simulink model "BLDC_LADRC_Motor_Speed_Control"  (R2022b)
settings: Solver=ode4  StartTime=0.0  StopTime=2  FixedStep=1e-6  RelTol=1e-3
model workspace (MAT data in the model file):
  Ctrol_Mode = 1
  Current_Control_Mode = 2
  Current_PID_Upper_Limit = 1
  PWM_Period = 0.0001
  Speed_I = 10
  Speed_P = 10
  Speed_PID_Upper_Limit = 0.02
  Ts_time = 1e-06
  Wc = 1000
  Wo = 4000
  b0 = 300
  current_I = 1
  current_P = 100
  r = 80
undefined symbols (not defined in the file): sigbuilder_block
libraries: simulink x11, dsparch4 x6, spsSeriesRLCBranchLib x2, spsPermanentMagnetSynchronousMachineLib x1, spsCurrentMeasurementLib x1, spsDCVoltageSourceLib x1, slctrlblks x1, slpidlib x1, eePwmGenerator x1, spsTwoLevelConverterLib x1, spspowerguiLib x1
settings Model: Creator=31904  LastModifiedBy=31904

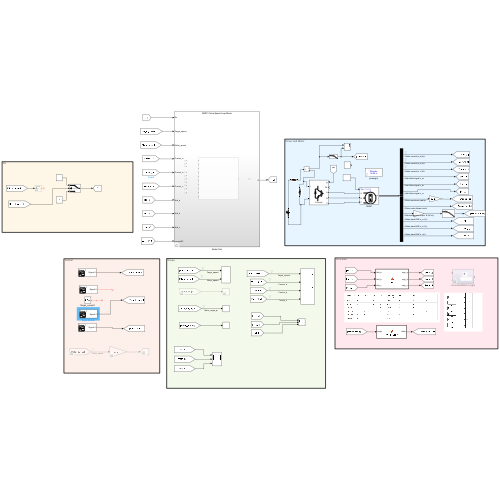
[thumbnail: Simulink's stored preview of the top-level diagram]
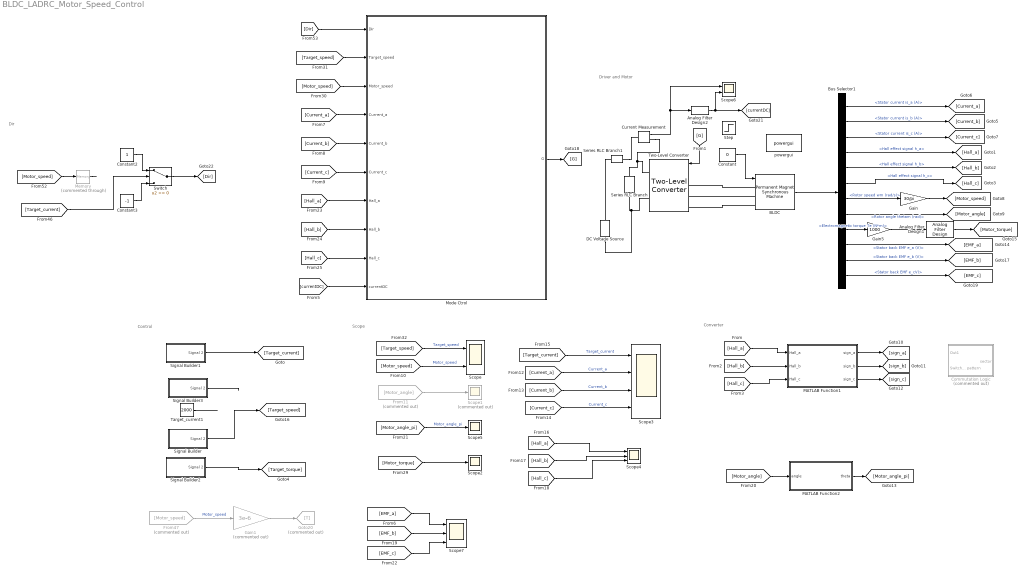
== system BLDC_LADRC_Motor_Speed_Control ==
  note: Dir
  note: Converter
  note: Control
  note: Scope
  note: Driver and Motor
  Analog Filter Design1 : dsparch4/Analog Filter Design  method=Butterworth  filttype=Lowpass  N=1  Wlo=1e2  Whi=80  Rp=2  Rs=40
  Analog Filter Design2 : dsparch4/Analog Filter Design  method=Butterworth  filttype=Lowpass  N=1  Wlo=100  Whi=80  Rp=2  Rs=40
  BLDC : spsPermanentMagnetSynchronousMachineLib/Permanent Magnet Synchronous Machine  NbPhases=3  FluxDistribution=Trapezoidal  RotorType=Round  MechanicalLoad=Torque Tm  PresetModel=No  ShowDetailedParameters=on  MeasurementBus=off  Resistance=1.005  Inductance=66e-6  dqInductances=[8.5e-3,8.5e-3]  La=0.0004  MachineConstant=Torque Constant (N.m / A_peak)  Flux=0.00785  VoltageCst=3.2882  TorqueCst=0.0314  Flat=120  Mechanical=[3e-05 0 2 0]  PolePairs=4  InitialConditions=[0,0, 0,0]  InitialConditions5ph=[0 0 0 0 0 0]  RefAngle=Aligned with phase A axis (original Park)  IterativeDiscreteModel=Trapezoidal non iterative  TsBlock=-1  TsPowergui=0
  Bus Selector1 : BusSelector  OutputSignals=Stator current is_a (A),Stator current is_b (A),Stator current is_c (A),Hall effect signal h_a,Hall effect signal h_b,Hall effect signal h_c,Rotor speed wm (rad/s),Rotor angle thetam (rad),Electromagnetic torque Te (N*m),Stator back EMF e_a (V),Stator back EMF e_b (V),Stator back EMF e_cV)
  Commutation Logic : Subsystem  Commented=on
  Constant : Constant  Value=0
  Constant2 : Constant
  Constant3 : Constant  Value=-1
  Current Measurement : spsCurrentMeasurementLib/Current Measurement  PhasorSimulation=off  OutputType=Complex  PSBequivalent=0
  DC Voltage Source : spsDCVoltageSourceLib/DC Voltage Source  Amplitude=28  Measurements=None
  From11 : From  Commented=on  GotoTag=Motor_angle
  From47 : From  Commented=on  GotoTag=Motor_speed
  Gain : Gain  Gain=30/pi
  Gain1 : Gain  Commented=on  Gain=3e-6
  Gain5 : Gain  Gain=1000
  Goto20 : Goto  Commented=on  GotoTag=T
  MATLAB Function1 : MATLAB Function  TreatAsAtomicUnit=on
  MATLAB Function2 : MATLAB Function  TreatAsAtomicUnit=on
  Memory : Memory  Commented=through
  Mode Ctrol : Subsystem  Variant=on
  Scope : Scope  NumInputPorts=2
  Scope1 : Scope  Commented=on
  Scope2 : Scope
  Scope3 : Scope  NumInputPorts=4
  Scope4 : Scope  NumInputPorts=3
  Scope5 : Scope
  Scope6 : Scope  NumInputPorts=2
  Scope7 : Scope  NumInputPorts=3
  Series RLC Branch : spsSeriesRLCBranchLib/Series RLC Branch  LConnTagsString=__new0  RConnTagsString=__new0  BranchType=C  Resistance=1  Inductance=1e-3  SetiL0=off  InitialCurrent=0  Capacitance=1e-6  Setx0=off  InitialVoltage=0  Measurements=None
  Series RLC Branch1 : spsSeriesRLCBranchLib/Series RLC Branch  LConnTagsString=__new0  RConnTagsString=__new0  BranchType=R  Resistance=1  Inductance=1e-3  SetiL0=off  InitialCurrent=0  Capacitance=1e-6  Setx0=off  InitialVoltage=0  Measurements=None
  Signal Builder : Subsystem  Tag=STV Subsys  LoadFcn=sigbuilder_block('load');  StartFcn=sigbuilder_block('start');  StopFcn=sigbuilder_block('stop');  ClipboardFcn=sigbuilder_block('clipboard');  mask(Sigbuilder block){tuvar=[0:10]}
      mask help: Simulink:masks:SigbuilderBlock_MD
      mask init:
      | if ~strcmp(get_param(bdroot(gcbh),'SimulationStatus'),'stopped') tuvar = sigbuilder_block('maskInit'); end
      settings: CopyFcn=sigbuilder_block('copy');  DeleteFcn=sigbuilder_block('delete');  ModelCloseFcn=sigbuilder_block('modelClose');  PreSaveFcn=sigbuilder_block('preSave');  PauseFcn=sigbuilder_block('pause');  ContinueFcn=sigbuilder_block('continue');  NameChangeFcn=sigbuilder_block('namechange');  OpenFcn=sigbuilder_block('open',[3234.3 -525.9 550.8 400.2 ]);  CloseFcn=sigbuilder_block('close');
      mask Display: plot(0, 0, 100, 100,[2, 2, 32, 32, 2], [68, 8, 8, 68, 68],[32, 2], [38, 38], [32, 19, 2],[53, 60, 44], [32, 17, 17, 2],[16, 16, 31, 31]);txt = getActiveGroup(gcbh);text(2, 100, txt,'verticalAlignment', 'top');
  Signal Builder1 : Subsystem  Tag=STV Subsys  LoadFcn=sigbuilder_block('load');  StartFcn=sigbuilder_block('start');  StopFcn=sigbuilder_block('stop');  ClipboardFcn=sigbuilder_block('clipboard');  mask(Sigbuilder block){tuvar=[0:10]}
      mask help: Simulink:masks:SigbuilderBlock_MD
      mask init:
      | if ~strcmp(get_param(bdroot(gcbh),'SimulationStatus'),'stopped') tuvar = sigbuilder_block('maskInit'); end
      settings: CopyFcn=sigbuilder_block('copy');  DeleteFcn=sigbuilder_block('delete');  ModelCloseFcn=sigbuilder_block('modelClose');  PreSaveFcn=sigbuilder_block('preSave');  PauseFcn=sigbuilder_block('pause');  ContinueFcn=sigbuilder_block('continue');  NameChangeFcn=sigbuilder_block('namechange');  OpenFcn=sigbuilder_block('open',[281.4 79.2 550.8 400.2 ]);  CloseFcn=sigbuilder_block('close');
      mask Display: plot(0, 0, 100, 100,[2, 2, 32, 32, 2], [68, 8, 8, 68, 68],[32, 2], [38, 38], [32, 19, 2],[53, 60, 44], [32, 17, 17, 2],[16, 16, 31, 31]);txt = getActiveGroup(gcbh);text(2, 100, txt,'verticalAlignment', 'top');
  Signal Builder2 : Subsystem  Tag=STV Subsys  LoadFcn=sigbuilder_block('load');  StartFcn=sigbuilder_block('start');  StopFcn=sigbuilder_block('stop');  ClipboardFcn=sigbuilder_block('clipboard');  mask(Sigbuilder block){tuvar=[0:10]}
      mask help: Simulink:masks:SigbuilderBlock_MD
      mask init:
      | if ~strcmp(get_param(bdroot(gcbh),'SimulationStatus'),'stopped') tuvar = sigbuilder_block('maskInit'); end
      settings: CopyFcn=sigbuilder_block('copy');  DeleteFcn=sigbuilder_block('delete');  ModelCloseFcn=sigbuilder_block('modelClose');  PreSaveFcn=sigbuilder_block('preSave');  PauseFcn=sigbuilder_block('pause');  ContinueFcn=sigbuilder_block('continue');  NameChangeFcn=sigbuilder_block('namechange');  OpenFcn=sigbuilder_block('open',[281.4 79.2 550.8 400.2 ]);  CloseFcn=sigbuilder_block('close');
      mask Display: plot(0, 0, 100, 100,[2, 2, 32, 32, 2], [68, 8, 8, 68, 68],[32, 2], [38, 38], [32, 19, 2],[53, 60, 44], [32, 17, 17, 2],[16, 16, 31, 31]);txt = getActiveGroup(gcbh);text(2, 100, txt,'verticalAlignment', 'top');
  Signal Builder3 : Subsystem  Tag=STV Subsys  LoadFcn=sigbuilder_block('load');  StartFcn=sigbuilder_block('start');  StopFcn=sigbuilder_block('stop');  ClipboardFcn=sigbuilder_block('clipboard');  mask(Sigbuilder block){tuvar=[0:10]}
      mask help: Simulink:masks:SigbuilderBlock_MD
      mask init:
      | if ~strcmp(get_param(bdroot(gcbh),'SimulationStatus'),'stopped') tuvar = sigbuilder_block('maskInit'); end
      settings: CopyFcn=sigbuilder_block('copy');  DeleteFcn=sigbuilder_block('delete');  ModelCloseFcn=sigbuilder_block('modelClose');  PreSaveFcn=sigbuilder_block('preSave');  PauseFcn=sigbuilder_block('pause');  ContinueFcn=sigbuilder_block('continue');  NameChangeFcn=sigbuilder_block('namechange');  OpenFcn=sigbuilder_block('open',[281.4 79.2 550.8 400.2 ]);  CloseFcn=sigbuilder_block('close');
      mask Display: plot(0, 0, 100, 100,[2, 2, 32, 32, 2], [68, 8, 8, 68, 68],[32, 2], [38, 38], [32, 19, 2],[53, 60, 44], [32, 17, 17, 2],[16, 16, 31, 31]);txt = getActiveGroup(gcbh);text(2, 100, txt,'verticalAlignment', 'top');
  Step : Step  Time=0  After=0.0005  SampleTime=0
  Switch : Switch  SaturateOnIntegerOverflow=off  InputSameDT=off
  Target_current1 : Constant  Value=2000
  Two-Level Converter : spsTwoLevelConverterLib/Two-Level Converter  ModelType=Switching devices  Ron=0.0001  Rs=1e6  Cs=inf  Vforward=[0,0]  Ron_Diode=1e-3  Rs_Diode=1e6  Cs_Diode=inf  Vf_Diode=1e-3  Rs_CurrentSource=inf  Ron_ACsource=1e-3
  powergui : spspowerguiLib/powergui  Priority=1  SimulationMode=Discrete  SampleTime=0.000001  frequency=60  Iterations=50  frequencyindice=0  Pbase=100e6  ErrMax=1e-4  UnitsV=kV  UnitsW=MW  buscounter=0  FunctionMessages=off  echomessages=off  EnableUseOfTLC=off  CurrentSourceSwitches=off  DisableSnubberDevices=off  DisableRonSwitches=off  DisableVfSwitches=off  DisplayEquations=off  AutomaticDiscreteSolvers=off  SolverType=Tustin/Backward Euler (TBE)  Interpol=off  ExternalGateDelay=off  methode=off  Ts=100  x0status=blocks  SPID=on  SwTol=0  HookPort=off  NonlinearTolerance=1e-4  nMaxIteration=100  ContinueOnMaxIteration=off  RestoreLinks=warning  ResistiveCurrentMeasurement=off  Frange=[0:2:500]  Ylog=off  Xlog=on  ShowGrid=off  save=off  variable=ZData  structure=0  ZoomFFT=off  StartTime=0.0  cycles=1  DisplayStyle=1  fundamental=60  FreqAxis=off  MaxFrequency=1000  frequencyindicesteady=1  RmsSteady=1  display=off
  wires:
  [G] -> Two-Level Converter/1
  Bus Selector1/3 -> [Current_c]  "<Stator current is_c (A)>"
  Bus Selector1/8 -> [Motor_angle]  "<Rotor angle thetam (rad)>"
  Bus Selector1/1 -> [Current_a]  "<Stator current is_a (A)>"
  Bus Selector1/6 -> [Hall_c]  "<Hall effect signal h_c>"
  Bus Selector1/4 -> [Hall_a]  "<Hall effect signal h_a>"
  Bus Selector1/2 -> [Current_b]  "<Stator current is_b (A)>"
  Bus Selector1/7 -> Gain/1  "<Rotor speed wm (rad/s)>"
  Bus Selector1/5 -> [Hall_b]  "<Hall effect signal h_b>"
  [Hall_a] -> MATLAB Function1/1(Hall_a)
  [Hall_b] -> MATLAB Function1/2(Hall_b)
  [Hall_c] -> MATLAB Function1/3(Hall_c)
  MATLAB Function1/1(sign_a) -> [sign_a]
  MATLAB Function1/2(sign_b) -> [sign_b]
  MATLAB Function1/3(sign_c) -> [sign_c]
  [Motor_speed] -> Scope/2  "Motor_speed"
  [Current_a] -> Scope3/2  "Current_a"
  [Current_b] -> Scope3/3  "Current_b"
  [Current_c] -> Scope3/4  "Current_c"
  [Target_current] -> Scope3/1  "Target_current"
  [Hall_a] -> Scope4/1
  [Hall_b] -> Scope4/2
  [Hall_c] -> Scope4/3
  From11/1 -> Scope1/1
  [Motor_angle] -> MATLAB Function2/1(angle)
  [Motor_angle_pi] -> Scope5/1  "Motor_angle_pi"
  MATLAB Function2/1(theta) -> [Motor_angle_pi]
  Bus Selector1/9 -> Gain5/1  "<Electromagnetic torque Te (N*m)>"
  [Motor_torque] -> Scope2/1
  [Target_speed] -> Scope/1  "Target_speed"
  Mode Ctrol/1(G) -> [G]
  [Target_speed] -> Mode Ctrol/2(Target_speed)
  [Motor_speed] -> Mode Ctrol/3(Motor_speed)
  [Current_a] -> Mode Ctrol/4(Current_a)
  [Current_b] -> Mode Ctrol/5(Current_b)
  [Current_c] -> Mode Ctrol/6(Current_c)
  Gain/1 -> [Motor_speed]
  Bus Selector1/10 -> [EMF_a]  "<Stator back EMF e_a (V)>"
  Bus Selector1/11 -> [EMF_b]  "<Stator back EMF e_b (V)>"
  Bus Selector1/12 -> [EMF_c]  "<Stator back EMF e_cV)>"
  [EMF_a] -> Scope7/1
  [EMF_b] -> Scope7/2
  [EMF_c] -> Scope7/3
  [Hall_a] -> Mode Ctrol/7(Hall_a)
  [Hall_b] -> Mode Ctrol/8(Hall_b)
  [Hall_c] -> Mode Ctrol/9(Hall_c)
  From47/1 -> Gain1/1  "Motor_speed"
  Gain1/1 -> Goto20/1
  BLDC/1 -> Bus Selector1/1
  Constant2/1 -> Switch/1
  Constant3/1 -> Switch/3
  Switch/1 -> [Dir]
  [Dir] -> Mode Ctrol/1(Dir)
  Gain5/1 -> Analog Filter Design1/1
  Signal Builder/1(Signal 2) -> [Target_speed]
  Constant/1 -> BLDC/1
  Current Measurement/1 -> Scope6/1, Analog Filter Design2/1
  Analog Filter Design2/1 -> [currentDC], Scope6/2
  [currentDC] -> Mode Ctrol/10(currentDC)
  [Motor_speed] -> Memory/1
  Memory/1 -> ?
  [Target_current] -> Switch/2
  Signal Builder1/1(Signal 2) -> [Target_current]
  Analog Filter Design1/1 -> [Motor_torque]
  Signal Builder2/1(Signal 2) -> [Target_torque]
  Target_current1/1 -> ?
  Signal Builder3/1(Signal 2) -> ?
  connections:
  DC Voltage Source/LConn1 -- Series RLC Branch/RConn1 -- Two-Level Converter/RConn2
  BLDC/LConn1 -- Two-Level Converter/LConn1
  BLDC/LConn2 -- Two-Level Converter/LConn2
  BLDC/LConn3 -- Two-Level Converter/LConn3
  Current Measurement/RConn1 -- Series RLC Branch/LConn1 -- Two-Level Converter/RConn1
  Series RLC Branch1/LConn1 -- DC Voltage Source/RConn1
  Series RLC Branch1/RConn1 -- Current Measurement/LConn1

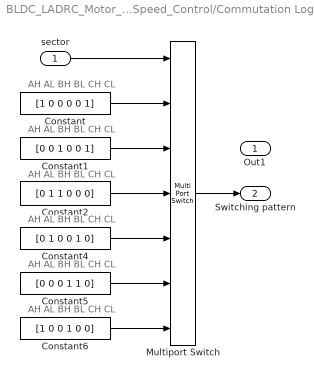
== system BLDC_LADRC_Motor_Speed_Control/Commutation Logic ==
  note: AH AL BH BL CH CL
  note: AH AL BH BL CH CL
  note: AH AL BH BL CH CL
  note: AH AL BH BL CH CL
  note: AH AL BH BL CH CL
  note: AH AL BH BL CH CL
  sector : Inport
  Constant : Constant  Value=[1 0 0 0 0 1]
  Constant1 : Constant  Value=[0 0 1 0 0 1]
  Constant2 : Constant  Value=[0 1 1 0 0 0]
  Constant4 : Constant  Value=[0 1 0 0 1 0]
  Constant5 : Constant  Value=[0 0 0 1 1 0]
  Constant6 : Constant  Value=[1 0 0 1 0 0]
  Multiport Switch : MultiPortSwitch  Inputs=6  SaturateOnIntegerOverflow=off  InputSameDT=off
  Out1 : Outport
  "  Switching pattern" : Outport  Port=2  VectorParamsAs1DForOutWhenUnconnected=off
  wires:
  Constant4/1 -> Multiport Switch/5
  Constant5/1 -> Multiport Switch/6
  Constant6/1 -> Multiport Switch/7
  sector/1 -> Multiport Switch/1
  Constant2/1 -> Multiport Switch/4
  Multiport Switch/1 -> "  Switching pattern"/1
  Constant1/1 -> Multiport Switch/3
  Constant/1 -> Multiport Switch/2

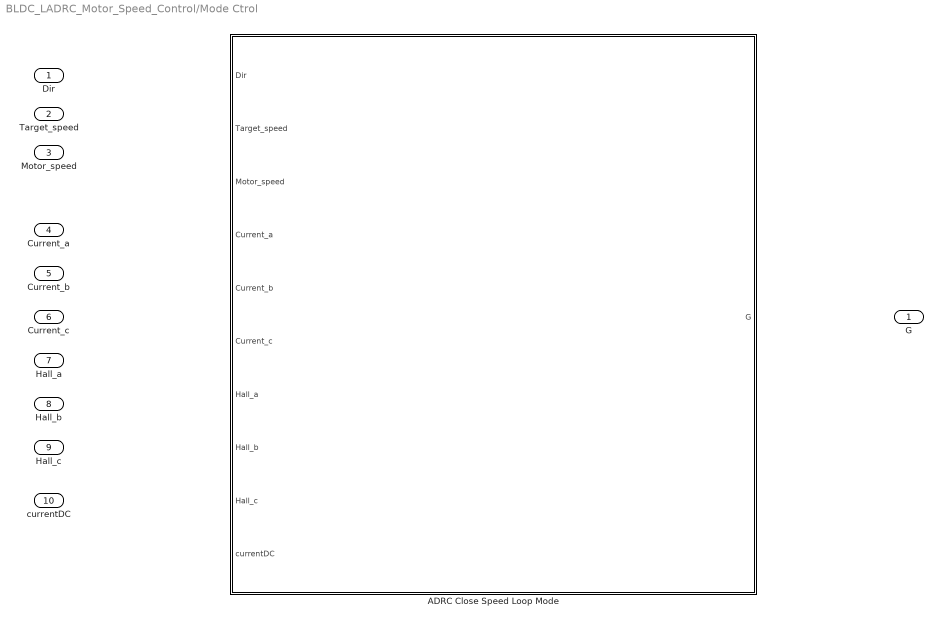
== system BLDC_LADRC_Motor_Speed_Control/Mode Ctrol ==
  Dir : Inport
  Target_speed : Inport  Port=2
  Motor_speed : Inport  Port=3
  Current_a : Inport  Port=4
  Current_b : Inport  Port=5
  Current_c : Inport  Port=6
  Hall_a : Inport  Port=7
  Hall_b : Inport  Port=8
  Hall_c : Inport  Port=9
  currentDC : Inport  Port=10
  ADRC Close Speed Loop Mode : Subsystem  TreatAsAtomicUnit=on  VariantControl=Ctrol_Mode==1
  G : Outport

== system BLDC_LADRC_Motor_Speed_Control/Signal Builder ==
  Demux : Demux  Tag=STV Demux  Outputs=1
      settings: DisplayOption=none
  FromWs : FromWorkspace  Tag=STV FromWs  VariableName=tuvar
      SigBuilderData=|
      | common.afterFinalStr = 'Extrapolate'
      | common.sampleTime = 0
      | dataSet.timeRange = [0 2]
      | dataSet.name = 'Group 1'
      | sbobj.Groups.Name = 'Group 1'
      | sbobj.Groups.Signals.Name = 'Signal 2'
      | sbobj.Groups.Signals.XData = [0 0.4 0.4 0.8 0.8 1.2 1.2 1.6 1.6 2]
      | sbobj.Groups.Signals.YData = [1000 1000 220 220 2000 2000 0 0 3000 3000]
      | sbobj.Groups.TimeRange = [0 2]
  Signal 2 : Outport  Tag=STV Outport
  wires:
  FromWs/1 -> Demux/1
  Demux/1 -> Signal 2/1

== system BLDC_LADRC_Motor_Speed_Control/Signal Builder1 ==
  Demux : Demux  Tag=STV Demux  Outputs=1
      settings: DisplayOption=none
  FromWs : FromWorkspace  Tag=STV FromWs  VariableName=tuvar
      SigBuilderData=|
      | common.afterFinalStr = 'Extrapolate'
      | common.sampleTime = 0
      | dataSet.timeRange = [0 10]
      | dataSet.name = 'Group 1'
      | sbobj.Groups.Name = 'Group 1'
      | sbobj.Groups.Signals.Name = 'Signal 2'
      | sbobj.Groups.Signals.XData = [0 0.2 0.2 0.4 0.4 10]
      | sbobj.Groups.Signals.YData = [1 1 -1 -1 0 0]
      | sbobj.Groups.TimeRange = [0 10]
  Signal 2 : Outport  Tag=STV Outport
  wires:
  Demux/1 -> Signal 2/1
  FromWs/1 -> Demux/1

== system BLDC_LADRC_Motor_Speed_Control/Signal Builder2 ==
  Demux : Demux  Tag=STV Demux  Outputs=1
      settings: DisplayOption=none
  FromWs : FromWorkspace  Tag=STV FromWs  VariableName=tuvar
      SigBuilderData=|
      | common.afterFinalStr = 'Extrapolate'
      | common.sampleTime = 0
      | dataSet.timeRange = [0 10]
      | dataSet.name = 'Group 1'
      | sbobj.Groups.Name = 'Group 1'
      | sbobj.Groups.Signals.Name = 'Signal 2'
      | sbobj.Groups.Signals.XData = [0 0.2 0.2 0.4 0.4 0.6 10]
      | sbobj.Groups.Signals.YData = [10 10 -10 -10 0 0 0]
      | sbobj.Groups.TimeRange = [0 10]
  Signal 2 : Outport  Tag=STV Outport
  wires:
  Demux/1 -> Signal 2/1
  FromWs/1 -> Demux/1

== system BLDC_LADRC_Motor_Speed_Control/Signal Builder3 ==
  Demux : Demux  Tag=STV Demux  Outputs=1
      settings: DisplayOption=none
  FromWs : FromWorkspace  Tag=STV FromWs  VariableName=tuvar
      SigBuilderData=|
      | common.afterFinalStr = 'Extrapolate'
      | common.sampleTime = 0
      | dataSet.timeRange = [0 0.5]
      | dataSet.name = 'Group 1'
      | sbobj.Groups.Name = 'Group 1'
      | sbobj.Groups.Signals.Name = 'Signal 2'
      | sbobj.Groups.Signals.XData = [0 0.1 0.4 0.5]
      | sbobj.Groups.Signals.YData = [1000 1000 -90 -100]
      | sbobj.Groups.TimeRange = [0 0.5]
  Signal 2 : Outport  Tag=STV Outport
  wires:
  Demux/1 -> Signal 2/1
  FromWs/1 -> Demux/1

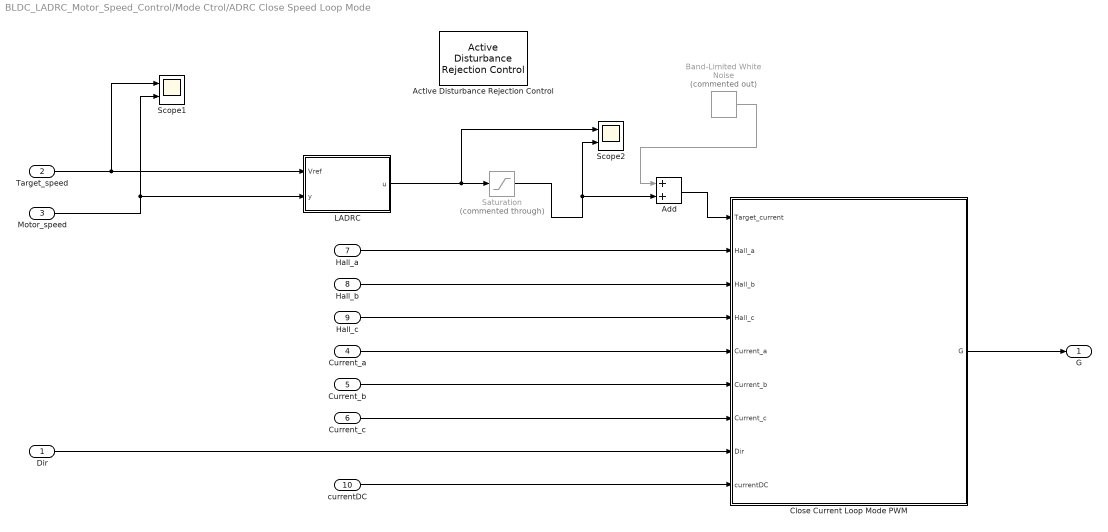
== system BLDC_LADRC_Motor_Speed_Control/Mode Ctrol/ADRC Close Speed Loop Mode ==
  Dir : Inport
  Target_speed : Inport  Port=2
  Motor_speed : Inport  Port=3
  Current_a : Inport  Port=4
  Current_b : Inport  Port=5
  Current_c : Inport  Port=6
  Hall_a : Inport  Port=7
  Hall_b : Inport  Port=8
  Hall_c : Inport  Port=9
  currentDC : Inport  Port=10
  Active Disturbance Rejection Control : slctrlblks/Active Disturbance Rejection Control  time_domain=discrete-time  Ts=0.00001  model_type=first-order  b0=100  wc=400  wo=1000  x0=0  ulim_checkbox=on  umax=20  umin=-20  xhat_checkbox=off
  Add : Sum
  Band-Limited White Noise : simulink/Sources/Band-Limited White Noise  Commented=on  Cov=[2]  Ts=1e-5  seed=[23341]
  Close Current Loop Mode PWM : Subsystem  TreatAsAtomicUnit=on  VariantControl=Ctrol_Mode==5
  LADRC : Subsystem
  Saturation : Saturate  Commented=through  UpperLimit=4  LowerLimit=-4
  Scope1 : Scope  NumInputPorts=2
  Scope2 : Scope  NumInputPorts=2
  G : Outport
  wires:
  Target_speed/1 -> LADRC/1(Vref), Scope1/1
  currentDC/1 -> Close Current Loop Mode PWM/9(currentDC)
  Dir/1 -> Close Current Loop Mode PWM/8(Dir)
  Motor_speed/1 -> LADRC/2(y), Scope1/2
  Hall_c/1 -> Close Current Loop Mode PWM/4(Hall_c)
  Hall_b/1 -> Close Current Loop Mode PWM/3(Hall_b)
  Hall_a/1 -> Close Current Loop Mode PWM/2(Hall_a)
  Close Current Loop Mode PWM/1(G) -> G/1
  Current_b/1 -> Close Current Loop Mode PWM/6(Current_b)
  Current_c/1 -> Close Current Loop Mode PWM/7(Current_c)
  Current_a/1 -> Close Current Loop Mode PWM/5(Current_a)
  LADRC/1(u) -> Scope2/1, Saturation/1
  Saturation/1 -> Scope2/2, Add/2
  Band-Limited White Noise/1 -> Add/1
  Add/1 -> Close Current Loop Mode PWM/1(Target_current)

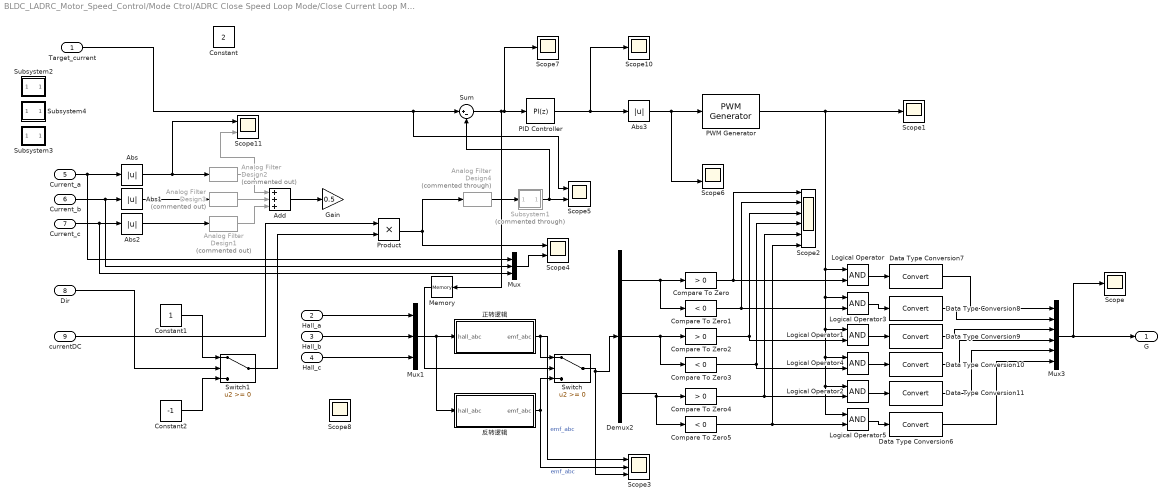
== system BLDC_LADRC_Motor_Speed_Control/Mode Ctrol/ADRC Close Speed Loop Mode/Close Current Loop Mode PWM ==
  Target_current : Inport
  Hall_a : Inport  Port=2
  Hall_b : Inport  Port=3
  Hall_c : Inport  Port=4
  Current_a : Inport  Port=5
  Current_b : Inport  Port=6
  Current_c : Inport  Port=7
  Dir : Inport  Port=8
  currentDC : Inport  Port=9
  Abs{,1..3} (4 alike) : Abs  SaturateOnIntegerOverflow=off
  Add : Sum  Inputs=+++
  Analog Filter Design1 : dsparch4/Analog Filter Design  Commented=on  method=Butterworth  filttype=Lowpass  N=1  Wlo=5e2  Whi=80  Rp=2  Rs=40
  Analog Filter Design2 : dsparch4/Analog Filter Design  Commented=on  method=Butterworth  filttype=Lowpass  N=1  Wlo=5e2  Whi=80  Rp=2  Rs=40
  Analog Filter Design3 : dsparch4/Analog Filter Design  Commented=on  method=Butterworth  filttype=Lowpass  N=1  Wlo=5e2  Whi=80  Rp=2  Rs=40
  Analog Filter Design4 : dsparch4/Analog Filter Design  Commented=through  method=Butterworth  filttype=Lowpass  N=1  Wlo=5e4  Whi=80  Rp=2  Rs=40
  Compare To Zero : simulink/Logic and Bit Operations/Compare To Zero  relop=>  OutDataTypeStr=boolean  ZeroCross=off
  Compare To Zero1 : simulink/Logic and Bit Operations/Compare To Zero  relop=<  OutDataTypeStr=boolean  ZeroCross=off
  Compare To Zero2 : simulink/Logic and Bit Operations/Compare To Zero  relop=>  OutDataTypeStr=boolean  ZeroCross=off
  Compare To Zero3 : simulink/Logic and Bit Operations/Compare To Zero  relop=<  OutDataTypeStr=boolean  ZeroCross=off
  Compare To Zero4 : simulink/Logic and Bit Operations/Compare To Zero  relop=>  OutDataTypeStr=boolean  ZeroCross=off
  Compare To Zero5 : simulink/Logic and Bit Operations/Compare To Zero  relop=<  OutDataTypeStr=boolean  ZeroCross=off
  Constant : Constant  Value=2
  Constant1 : Constant
  Constant2 : Constant  Value=-1
  Data Type Conversion{6..11} (6 alike) : DataTypeConversion  SaturateOnIntegerOverflow=off  RndMeth=Floor
  Demux2 : Demux  Outputs=3
  Gain : Gain  Gain=0.5
  Logical Operator{,1..5} (6 alike) : Logic  AllPortsSameDT=off  OutDataTypeStr=boolean
  Memory : Memory
  Mux : Mux  Inputs=3
  Mux1 : Mux  Inputs=3
  Mux3 : Mux  Inputs=6
  PID Controller : slpidlib/PID Controller  Controller=PI  Form=Parallel  TimeDomain=Discrete-time  UseExternalTs=off  SampleTime=1e-5  IntegratorMethod=Forward Euler  FilterMethod=Forward Euler  ControllerParametersSource=internal  P=current_P  I=current_I  UseKiTs=off  D=0  N=100  UseFilter=on  TunerSelectOption=Transfer Function Based (PID Tuner App)  InitialConditionSource=internal  InitialConditionForIntegrator=0  InitialConditionForFilter=0  DifferentiatorICPrevScaledInput=0  ExternalReset=none  TrackingMode=off  Kt=1  LimitOutput=on  SatLimitsSource=internal  UpperSaturationLimit=1  LowerSaturationLimit=-1  LinearizeAsGain=off  AntiWindupMode=none  Kb=1  LimitIntegrator=on  UpperIntegratorSaturationLimit=2  LowerIntegratorSaturationLimit=-2  POutMin=[]  POutMax=[]  IOutMin=[]  IOutMax=[]  DOutMin=[]  DOutMax=[]  NOutMin=[]  NOutMax=[]  SumOutMin=[]  SumOutMax=[]  SaturationOutMin=[]  SaturationOutMax=[]  PParamMin=[]  PParamMax=[]  IParamMin=[]  IParamMax=[]  DParamMin=[]  DParamMax=[]  NParamMin=[]  NParamMax=[]  KbParamMin=[]  KbParamMax=[]  KtParamMin=[]  KtParamMax=[]  KbOutMin=[]  KbOutMax=[]  KtOutMin=[]  KtOutMax=[]  IntegratorOutMin=[]  IntegratorOutMax=[]  FilterOutMin=[]  FilterOutMax=[]  SumI1OutMin=[]  SumI1OutMax=[]  SumI2OutMin=[]  SumI2OutMax=[]  SumI3OutMin=[]  SumI3OutMax=[]  SumI4OutMin=[]  SumI4OutMax=[]  SumDOutMin=[]  SumDOutMax=[]  DifferentiatorOutMin=[]  DifferentiatorOutMax=[]  FilterDiffOutCoefMin=[]  FilterDiffOutCoefMax=[]  ReciprocalOutMin=[]  ReciprocalOutMax=[]  SumDenOutMin=[]  SumDenOutMax=[]  SumNumOutMin=[]  SumNumOutMax=[]  DivideOutMin=[]  DivideOutMax=[]  UdiffTsProdOutMin=[]  UdiffTsProdOutMax=[]  NTsProdOutMin=[]  NTsProdOutMax=[]  UintegralTsProdOutMin=[]  UintegralTsProdOutMax=[]  UngainTsProdOutMin=[]  UngainTsProdOutMax=[]  ClampingZeroOutDataTypeStr=Inherit: Inherit via back propagation  ClampingZeroOutMin=[]  ClampingZeroOutMax=[]  FilterDenConstantOutDataTypeStr=Inherit: Inherit via back propagation  FilterDenConstantOutMin=[]  FilterDenConstantOutMax=[]  PCopyOutDataTypeStr=Inherit: Inherit via back propagation  PCopyOutMin=[]  PCopyOutMax=[]  NCopyOutDataTypeStr=Inherit: Inherit via back propagation  NCopyOutMin=[]  NCopyOutMax=[]  IntegratorContinuousStateAttributes=''  IntegratorStateMustResolveToSignalObject=off  IntegratorRTWStateStorageClass=Auto  FilterContinuousStateAttributes=''  FilterStateMustResolveToSignalObject=off  FilterRTWStateStorageClass=Auto  ParallelPVariant=InternalParameters  IdealPVariant=Disabled  IVariant=InternalParameters  DVariant=Disabled  IntegratorVariant=Discrete  SatVariant=Enabled  AWVariant=Passthrough  PCopyVariant=Disabled  TRVariant=Disabled  FdbkBlocksVariant=Forward  IdealPFdbkVariant=Disabled  SatFdbkVariant=Disabled  DerivativeFilterVariant=Disabled  NVariant=Disabled  NCopyVariant=Disabled_SignalSpec  FilterICVariant=Disabled  IntegratorICVariant=InternalICs  ExternalResetVariant=Disabled  TRSumVariant=Passthrough  SumFdbkVariant=Disabled  SumVariant=Sum_PI  TsampFilterVariant=InternalTs  TsampNgainVariant=Passthrough  TsampIntegralVariant=Passthrough  ExternalSaturationOutDataTypeStr=Inherit: Same as second input
  PWM Generator : eePwmGenerator/PWM Generator  CarrCount=Up  Tper=PWM_Period  Tdelay=0  Ts=Ts_time
  Product : Product
  Scope{,1,7..8,10} (5 alike) : Scope
  Scope{4..6,11} (4 alike) : Scope  NumInputPorts=2
  Scope2 : Scope  NumInputPorts=6
  Scope3 : Scope  NumInputPorts=3
  Subsystem1 : Subsystem  Commented=through
  Subsystem2 : Subsystem
  Subsystem3 : Subsystem
  Subsystem4 : Subsystem
  Sum : Sum  Inputs=|+-
  Switch : Switch  SaturateOnIntegerOverflow=off  InputSameDT=off
  Switch1 : Switch  SaturateOnIntegerOverflow=off  InputSameDT=off
  反转逻辑 : Subsystem
  正转逻辑 : Subsystem
  G : Outport
  wires:
  Analog Filter Design3/1 -> Add/2
  Abs/1 -> Scope11/1, Analog Filter Design2/1
  反转逻辑/1(emf_abc) -> Switch/3, Scope3/2  "emf_abc"
  Dir/1 -> Switch1/2
  Hall_c/1 -> Mux1/3
  Mux3/1 -> G/1, Scope/1
  Hall_a/1 -> Mux1/1
  Data Type Conversion9/1 -> Mux3/3
  Compare To Zero2/1 -> Scope2/3, Logical Operator1/2
  Constant1/1 -> Switch1/1
  Logical Operator5/1 -> Data Type Conversion6/1
  Data Type Conversion6/1 -> Mux3/6
  Memory/1 -> Switch/2
  currentDC/1 -> Product/1
  Compare To Zero4/1 -> Scope2/5, Logical Operator2/2
  Data Type Conversion11/1 -> Mux3/5
  Current_c/1 -> Abs2/1, Mux/3
  Product/1 -> Analog Filter Design4/1, Scope4/1
  Add/1 -> Gain/1
  Subsystem1/1(Out1) -> Sum/2, Scope5/2
  Logical Operator4/1 -> Data Type Conversion10/1
  Compare To Zero3/1 -> Logical Operator4/2, Scope2/4
  Data Type Conversion7/1 -> Mux3/1
  Abs2/1 -> Analog Filter Design1/1
  Hall_b/1 -> Mux1/2
  Analog Filter Design4/1 -> Subsystem1/1(In1)
  Analog Filter Design1/1 -> Add/3
  Constant2/1 -> Switch1/3
  Compare To Zero5/1 -> Scope2/6, Logical Operator5/2
  Data Type Conversion10/1 -> Mux3/4
  Sum/1 -> PID Controller/1, Scope7/1, Memory/1
  Logical Operator1/1 -> Data Type Conversion9/1
  PWM Generator/1 -> Scope1/1, Logical Operator2/1, Logical Operator5/1, Logical Operator4/1, Logical Operator1/1, Logical Operator3/1, Logical Operator/1
  Abs3/1 -> Scope6/2, PWM Generator/1
  Analog Filter Design2/1 -> Add/1, Scope11/2
  Compare To Zero/1 -> Scope2/1, Logical Operator/2
  Current_a/1 -> Mux/1, Abs/1
  Switch/1 -> Demux2/1, Scope3/3
  Abs1/1 -> Analog Filter Design3/1
  正转逻辑/1(emf_abc) -> Switch/1, Scope3/1  "emf_abc"
  Mux1/1 -> 反转逻辑/1(hall_abc), 正转逻辑/1(hall_abc)
  PID Controller/1 -> Abs3/1, Scope10/1
  Current_b/1 -> Abs1/1, Mux/2
  Logical Operator2/1 -> Data Type Conversion11/1
  Compare To Zero1/1 -> Scope2/2, Logical Operator3/2
  Target_current/1 -> Sum/1, Scope5/1
  Mux/1 -> Scope4/2
  Logical Operator/1 -> Data Type Conversion7/1
  Demux2/3 -> Compare To Zero4/1, Compare To Zero5/1
  Logical Operator3/1 -> Data Type Conversion8/1
  Demux2/2 -> Compare To Zero2/1, Compare To Zero3/1
  Data Type Conversion8/1 -> Mux3/2
  Demux2/1 -> Compare To Zero/1, Compare To Zero1/1
  Switch1/1 -> Product/2

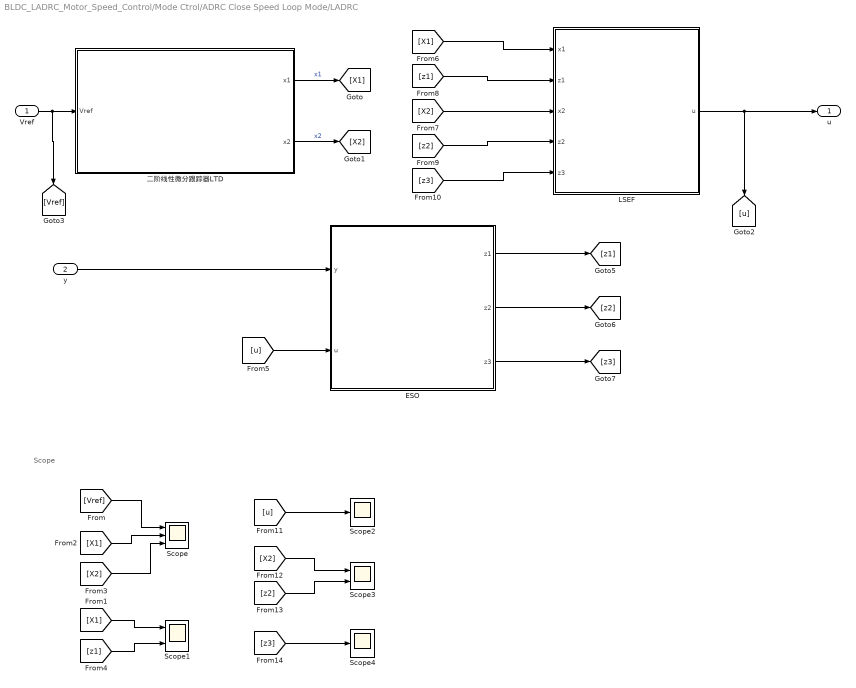
== system BLDC_LADRC_Motor_Speed_Control/Mode Ctrol/ADRC Close Speed Loop Mode/LADRC ==
  note: Scope
  Vref : Inport
  y : Inport  Port=2
  ESO : Subsystem
  LSEF : Subsystem
  Scope : Scope  NumInputPorts=3
  Scope1 : Scope  NumInputPorts=2
  Scope2 : Scope
  Scope3 : Scope  NumInputPorts=2
  Scope4 : Scope
  二阶线性微分跟踪器LTD : Subsystem
  u : Outport
  wires:
  [z2] -> LSEF/4(z2)
  [z3] -> LSEF/5(z3)
  [X1] -> LSEF/1(x1)
  ESO/1(z1) -> [z1]
  二阶线性微分跟踪器LTD/1(x1) -> [X1]  "x1"
  ESO/3(z3) -> [z3]
  y/1 -> ESO/1(y)
  二阶线性微分跟踪器LTD/2(x2) -> [X2]  "x2"
  ESO/2(z2) -> [z2]
  [u] -> ESO/2(u)
  [z1] -> LSEF/2(z1)
  [X2] -> LSEF/3(x2)
  Vref/1 -> [Vref], 二阶线性微分跟踪器LTD/1(Vref)
  LSEF/1(u) -> u/1, [u]
  [X1] -> Scope/2
  [Vref] -> Scope/1
  [X2] -> Scope/3
  [X1] -> Scope1/1
  [z1] -> Scope1/2
  [u] -> Scope2/1
  [X2] -> Scope3/1
  [z2] -> Scope3/2
  [z3] -> Scope4/1

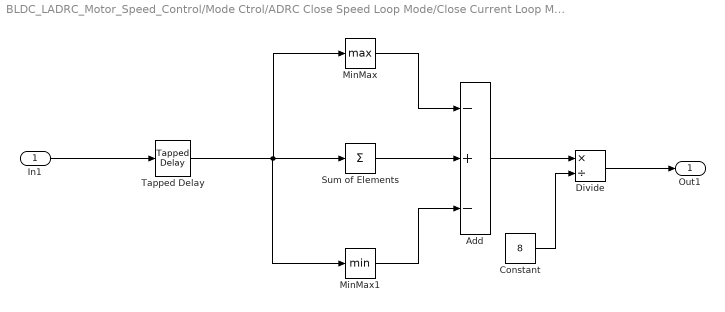
== system BLDC_LADRC_Motor_Speed_Control/Mode Ctrol/ADRC Close Speed Loop Mode/Close Current Loop Mode PWM/Subsystem1 ==
  In1 : Inport
  Add : Sum  Inputs=-+-
  Constant : Constant  Value=8
  Divide : Product  Inputs=*/
  MinMax : MinMax  Function=max
  MinMax1 : MinMax
  Sum of Elements : Sum  Inputs=+
  Tapped Delay : simulink/Discrete/Tapped Delay  vinit=0  samptime=-1  NumDelays=10  DelayOrder=Oldest  includeCurrent=off
  Out1 : Outport
  wires:
  In1/1 -> Tapped Delay/1
  Tapped Delay/1 -> MinMax1/1, MinMax/1, Sum of Elements/1
  MinMax/1 -> Add/1
  Sum of Elements/1 -> Add/2
  MinMax1/1 -> Add/3
  Add/1 -> Divide/1
  Constant/1 -> Divide/2
  Divide/1 -> Out1/1

== system BLDC_LADRC_Motor_Speed_Control/Mode Ctrol/ADRC Close Speed Loop Mode/Close Current Loop Mode PWM/Subsystem2 ==
  In1 : Inport
  Add : Sum  Inputs=-+-
  Constant : Constant  Value=998
  Divide : Product  Inputs=*/
  MinMax : MinMax  Function=max
  MinMax1 : MinMax
  Sum of Elements : Sum  Inputs=+
  Tapped Delay : simulink/Discrete/Tapped Delay  vinit=0  samptime=-1  NumDelays=1000  DelayOrder=Oldest  includeCurrent=off
  Out1 : Outport
  wires:
  Divide/1 -> Out1/1
  Constant/1 -> Divide/2
  Add/1 -> Divide/1
  MinMax1/1 -> Add/3
  Sum of Elements/1 -> Add/2
  MinMax/1 -> Add/1
  Tapped Delay/1 -> Sum of Elements/1, MinMax/1, MinMax1/1
  In1/1 -> Tapped Delay/1

== system BLDC_LADRC_Motor_Speed_Control/Mode Ctrol/ADRC Close Speed Loop Mode/Close Current Loop Mode PWM/Subsystem3 ==
  In1 : Inport
  Add : Sum  Inputs=-+-
  Constant : Constant  Value=998
  Divide : Product  Inputs=*/
  MinMax : MinMax  Function=max
  MinMax1 : MinMax
  Sum of Elements : Sum  Inputs=+
  Tapped Delay : simulink/Discrete/Tapped Delay  vinit=0  samptime=-1  NumDelays=1000  DelayOrder=Oldest  includeCurrent=off
  Out1 : Outport
  wires:
  In1/1 -> Tapped Delay/1
  Tapped Delay/1 -> MinMax1/1, MinMax/1, Sum of Elements/1
  MinMax/1 -> Add/1
  Sum of Elements/1 -> Add/2
  MinMax1/1 -> Add/3
  Add/1 -> Divide/1
  Constant/1 -> Divide/2
  Divide/1 -> Out1/1

== system BLDC_LADRC_Motor_Speed_Control/Mode Ctrol/ADRC Close Speed Loop Mode/Close Current Loop Mode PWM/Subsystem4 ==
  In1 : Inport
  Add : Sum  Inputs=-+-
  Constant : Constant  Value=998
  Divide : Product  Inputs=*/
  MinMax : MinMax  Function=max
  MinMax1 : MinMax
  Sum of Elements : Sum  Inputs=+
  Tapped Delay : simulink/Discrete/Tapped Delay  vinit=0  samptime=-1  NumDelays=1000  DelayOrder=Oldest  includeCurrent=off
  Out1 : Outport
  wires:
  Divide/1 -> Out1/1
  Constant/1 -> Divide/2
  Add/1 -> Divide/1
  MinMax1/1 -> Add/3
  Sum of Elements/1 -> Add/2
  MinMax/1 -> Add/1
  Tapped Delay/1 -> Sum of Elements/1, MinMax/1, MinMax1/1
  In1/1 -> Tapped Delay/1

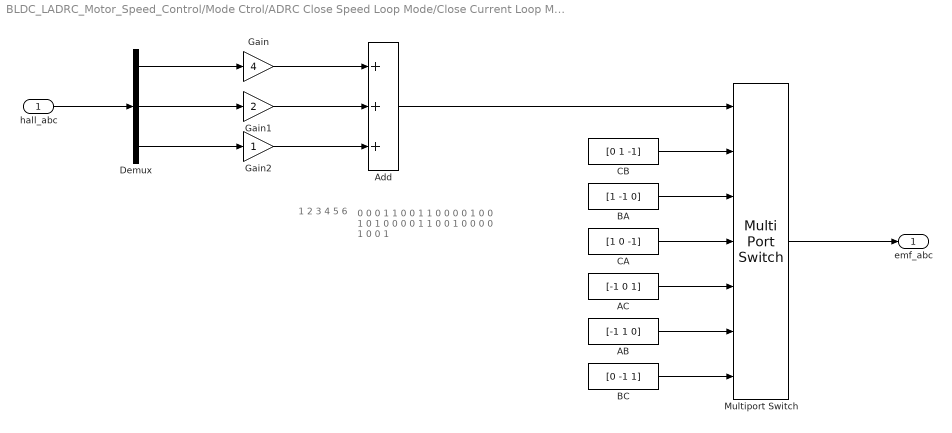
== system BLDC_LADRC_Motor_Speed_Control/Mode Ctrol/ADRC Close Speed Loop Mode/Close Current Loop Mode PWM/反转逻辑 ==
  note: 1
      | 2
      | 3
      | 4
      | 5
      | 6
  note: 0 0 0 1 1 0
      | 0 1 1 0 0 0
      | 0 1 0 0 1 0
      | 1 0 0 0 0 1
      | 1 0 0 1 0 0
      | 0 0 1 0 0 1
  hall_abc : Inport
  AB : Constant  Value=[-1 1 0]
  AC : Constant  Value=[-1 0 1]
  Add : Sum  Inputs=+++
  BA : Constant  Value=[1 -1 0]
  BC : Constant  Value=[0 -1 1]
  CA : Constant  Value=[1 0 -1]
  CB : Constant  Value=[0 1 -1]
  Demux : Demux  Outputs=3
  Gain : Gain  Gain=4
  Gain1 : Gain  Gain=2
  Gain2 : Gain
  Multiport Switch : MultiPortSwitch  Inputs=6  DiagnosticForDefault=None  SaturateOnIntegerOverflow=off  InputSameDT=off
  emf_abc : Outport
  wires:
  hall_abc/1 -> Demux/1
  Demux/3 -> Gain2/1
  Demux/1 -> Gain/1
  Demux/2 -> Gain1/1
  Gain2/1 -> Add/3
  Gain1/1 -> Add/2
  Gain/1 -> Add/1
  AC/1 -> Multiport Switch/5
  Add/1 -> Multiport Switch/1
  Multiport Switch/1 -> emf_abc/1
  BC/1 -> Multiport Switch/7
  AB/1 -> Multiport Switch/6
  CA/1 -> Multiport Switch/4
  CB/1 -> Multiport Switch/2
  BA/1 -> Multiport Switch/3

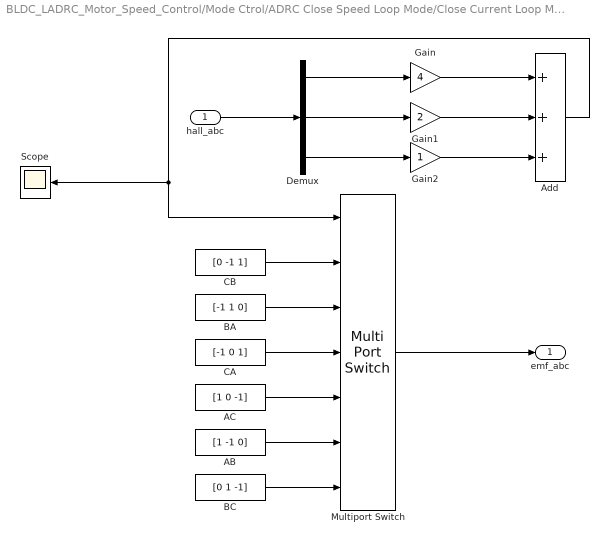
== system BLDC_LADRC_Motor_Speed_Control/Mode Ctrol/ADRC Close Speed Loop Mode/Close Current Loop Mode PWM/正转逻辑 ==
  hall_abc : Inport
  AB : Constant  Value=[1 -1 0]
  AC : Constant  Value=[1 0 -1]
  Add : Sum  Inputs=+++
  BA : Constant  Value=[-1 1 0]
  BC : Constant  Value=[0 1 -1]
  CA : Constant  Value=[-1 0 1]
  CB : Constant  Value=[0 -1 1]
  Demux : Demux  Outputs=3
  Gain : Gain  Gain=4
  Gain1 : Gain  Gain=2
  Gain2 : Gain
  Multiport Switch : MultiPortSwitch  Inputs=6  DiagnosticForDefault=None  SaturateOnIntegerOverflow=off  InputSameDT=off
  Scope : Scope
  emf_abc : Outport
  wires:
  hall_abc/1 -> Demux/1
  Demux/3 -> Gain2/1
  Demux/1 -> Gain/1
  Demux/2 -> Gain1/1
  Gain2/1 -> Add/3
  Gain1/1 -> Add/2
  Gain/1 -> Add/1
  AC/1 -> Multiport Switch/5
  Add/1 -> Multiport Switch/1, Scope/1
  Multiport Switch/1 -> emf_abc/1
  BC/1 -> Multiport Switch/7
  AB/1 -> Multiport Switch/6
  CA/1 -> Multiport Switch/4
  CB/1 -> Multiport Switch/2
  BA/1 -> Multiport Switch/3

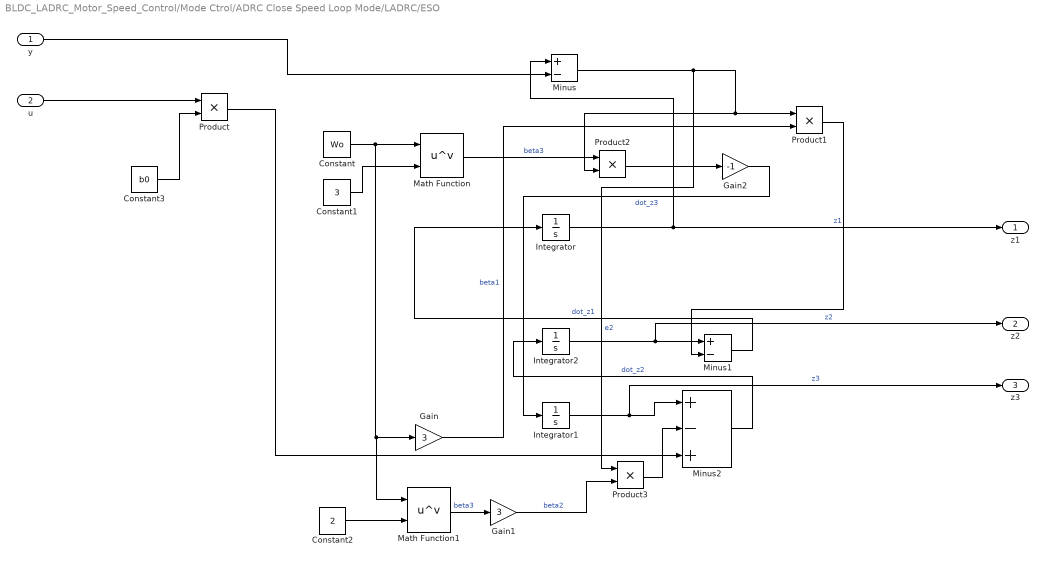
== system BLDC_LADRC_Motor_Speed_Control/Mode Ctrol/ADRC Close Speed Loop Mode/LADRC/ESO ==
  y : Inport
  u : Inport  Port=2
  Constant : Constant  Value=Wo
  Constant1 : Constant  Value=3
  Constant2 : Constant  Value=2
  Constant3 : Constant  Value=b0
  Gain : Gain  Gain=3
  Gain1 : Gain  Gain=3
  Gain2 : Gain  Gain=-1
  Integrator : Integrator
  Integrator1 : Integrator
  Integrator2 : Integrator
  Math Function : Math  Operator=pow
  Math Function1 : Math  Operator=pow
  Minus : Sum  Inputs=+-
  Minus1 : Sum  Inputs=+-
  Minus2 : Sum  Inputs=+-+
  Product{,1..3} (4 alike) : Product
  z1 : Outport
  z2 : Outport  Port=2
  z3 : Outport  Port=3
  wires:
  y/1 -> Minus/2
  Minus/1 -> Product3/1, Product2/2, Product1/1  "e2"
  Math Function1/1 -> Gain1/1  "beta3"
  Math Function/1 -> Product2/1  "beta3"
  Constant/1 -> Math Function/1, Math Function1/1, Gain/1
  Gain/1 -> Product1/2  "beta1"
  Product/1 -> Minus2/3
  Integrator2/1 -> z2/1, Minus1/1  "z2"
  Integrator/1 -> z1/1, Minus/1  "z1"
  Product1/1 -> Minus1/2
  Constant1/1 -> Math Function/2
  Constant2/1 -> Math Function1/2
  Product2/1 -> Gain2/1
  Integrator1/1 -> z3/1, Minus2/1  "z3"
  Gain1/1 -> Product3/2  "beta2"
  Minus1/1 -> Integrator/1  "dot_z1"
  Gain2/1 -> Integrator1/1  "dot_z3"
  Product3/1 -> Minus2/2
  Constant3/1 -> Product/2
  u/1 -> Product/1
  Minus2/1 -> Integrator2/1  "dot_z2"

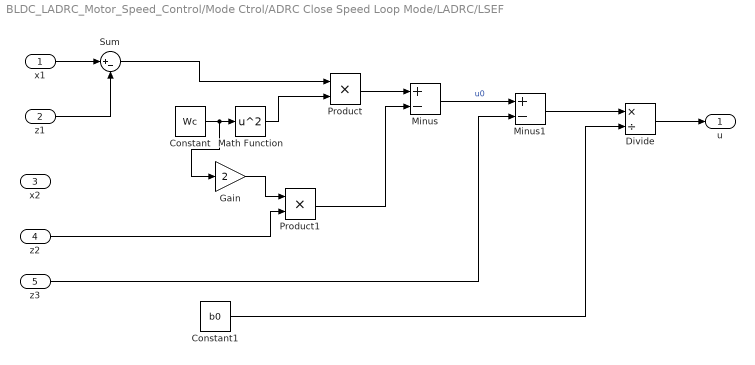
== system BLDC_LADRC_Motor_Speed_Control/Mode Ctrol/ADRC Close Speed Loop Mode/LADRC/LSEF ==
  x1 : Inport
  z1 : Inport  Port=2
  x2 : Inport  Port=3
  z2 : Inport  Port=4
  z3 : Inport  Port=5
  Constant : Constant  Value=Wc
  Constant1 : Constant  Value=b0
  Divide : Product  Inputs=*/
  Gain : Gain  Gain=2
  Math Function : Math  Operator=square
  Minus : Sum  Inputs=+-
  Minus1 : Sum  Inputs=+-
  Product : Product
  Product1 : Product
  Sum : Sum  Inputs=|+-
  u : Outport
  wires:
  Math Function/1 -> Product/2
  Sum/1 -> Product/1
  Constant/1 -> Gain/1, Math Function/1
  z2/1 -> Product1/2
  x1/1 -> Sum/1
  Product1/1 -> Minus/2
  Minus/1 -> Minus1/1  "u0"
  Gain/1 -> Product1/1
  Product/1 -> Minus/1
  z1/1 -> Sum/2
  z3/1 -> Minus1/2
  Minus1/1 -> Divide/1
  Constant1/1 -> Divide/2
  Divide/1 -> u/1

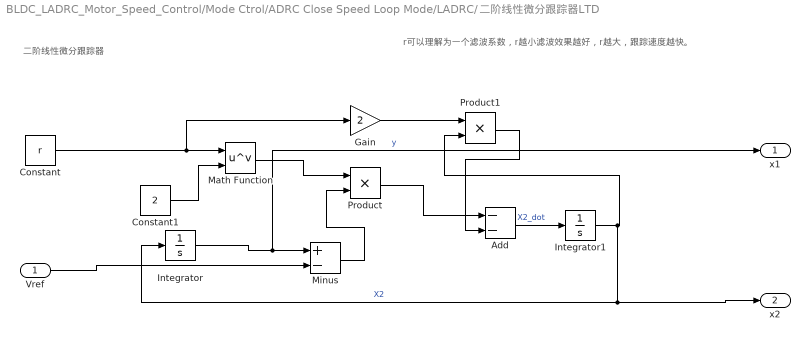
== system BLDC_LADRC_Motor_Speed_Control/Mode Ctrol/ADRC Close Speed Loop Mode/LADRC/二阶线性微分跟踪器LTD ==
  note: r可以理解为一个滤波系数，r越小滤波效果越好，r越大，跟踪速度越快。
  note: 二阶线性微分跟踪器
  Vref : Inport
  Add : Sum  Inputs=--
  Constant : Constant  Value=r
  Constant1 : Constant  Value=2
  Gain : Gain  Gain=2
  Integrator : Integrator
  Integrator1 : Integrator
  Math Function : Math  Operator=pow
  Minus : Sum  Inputs=+-
  Product : Product
  Product1 : Product
  x1 : Outport
  x2 : Outport  Port=2
  wires:
  Constant/1 -> Gain/1, Math Function/1
  Integrator/1 -> x1/1, Minus/1  "y"
  Minus/1 -> Product/2
  Product/1 -> Add/1
  Math Function/1 -> Product/1
  Constant1/1 -> Math Function/2
  Integrator1/1 -> x2/1, Integrator/1, Product1/2  "X2"
  Gain/1 -> Product1/1
  Add/1 -> Integrator1/1  "X2_dot"
  Product1/1 -> Add/2
  Vref/1 -> Minus/2

== matlab function BLDC_LADRC_Motor_Speed_Control/MATLAB Function2 ==
  data: angle input; theta output
function theta = Angle_Conv(angle)

n=mod(angle,pi);

theta = n;

== matlab function BLDC_LADRC_Motor_Speed_Control/MATLAB Function1 ==
  data: Hall_a input; sign_a output; Hall_b input; Hall_c input; sign_b output; sign_c output
function [sign_a,sign_b,sign_c] = fcn(Hall_a, Hall_b, Hall_c)

if Hall_a==1&&Hall_b==0&&Hall_c==1

sign_a=1;
sign_b=0;
sign_c=-1;

elseif Hall_a==1&&Hall_b==0&&Hall_c==0

sign_a=0;
sign_b=1;
sign_c=-1;


elseif Hall_a==1&&Hall_b==1&&Hall_c==0

sign_a=-1;
sign_b=1;
sign_c=0;


elseif Hall_a==0&&Hall_b==1&&Hall_c==0

sign_a=-1;
sign_b=0;
sign_c=1;


elseif Hall_a==0&&Hall_b==1&&Hall_c==1

sign_a=0;
sign_b=-1;
sign_c=1;

else

sign_a=1;
sign_b=-1;
sign_c=0;


end
